simulink model "tricanter_top"  (R2025b)
settings: Solver=FixedStepDiscrete  StartTime=0  StopTime=1500  FixedStep=Ts  RelTol=1e-3
values from neighbouring files (symbols this model uses):
  m0 = 0.0 0.0 0.0 0.0 0.0 0.0 0.0 0.0 0.0 0.0 0.0 0.0 0.0 0.0 0.0 0.0 0.0 0.0 0.0 0.0 0.0 0.0 0.0 0.0 0.0    [tricanter_data.sldd]
  phi0 = 0.0 0.0 0.0 0.0 0.0 0.0 0.0 0.0 0.0 0.0 0.0 0.0 0.0 0.0 0.0 0.0 0.0 0.0 0.0 0.0 0.0 0.0 0.0 0.0 0.0 0.0 0.0 0.0 0.0 0.0 0.0 0.0 0.0 0.0 0.0 0.0 0.0 0.0 0.0 0.0 0.0 0.0 0.0 0.0 0.0 0.0 0.0 0.0 0.0 0.0 0.0 0.0 0.0 0.0 0.0 0.0 0.0 0.0 0.0 0.0 0.0 0.0 0.0 0.0 0.0 0.0 0.0 0.0 0.0 0.0 0.0 0.0 0.0 0.0 0.0 0.0 0.0 0.0 0.0 0.0 0.0 0.0 0.0 0.0 0.0 0.0 0.0 0.0 0.0 0.0 0.0 0.0 0.0 0.0 0.0 0.0 0.0 0.0 0.0 0.0    [tricanter_data.sldd]
  TricInputs0 = 0.03    [tricanter_data.sldd]
  TricParams = 0.04    [tricanter_data.sldd]
  Ts = 1.0    [tricanter_data.sldd]
undefined symbols (not defined in the file or in its folder): DiscIntNeverNeededParam
settings Model: DataDictionary=tricanter_data.sldd  Creator=User  LastModifiedBy=User

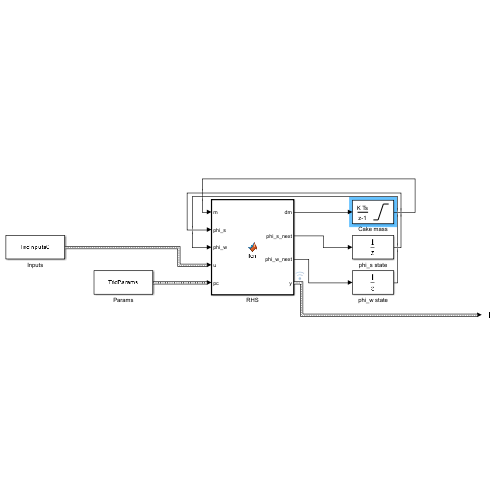
[thumbnail: Simulink's stored preview of the top-level diagram]
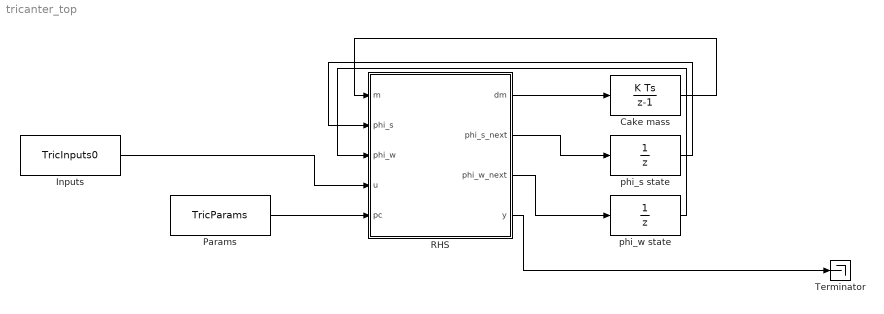
== system tricanter_top ==
  Cake mass : DiscreteIntegrator  InitialCondition=m0  SampleTime=Ts  LimitOutput=on  LowerSaturationLimit=0  ICPrevOutput=DiscIntNeverNeededParam  ICPrevScaledInput=DiscIntNeverNeededParam
  Inputs : Constant  Value=TricInputs0  VectorParams1D=off  OutDataTypeStr=Bus: BusTricInputs
  Params : Constant  Value=TricParams  VectorParams1D=off  OutDataTypeStr=Bus: BusTricParams
  RHS : MATLAB Function  TreatAsAtomicUnit=on
  Terminator : Terminator
  phi_s state : UnitDelay  InitialCondition=phi0  SampleTime=Ts  HasFrameUpgradeWarning=on
  phi_w state : UnitDelay  InitialCondition=phi0  SampleTime=Ts  HasFrameUpgradeWarning=on
  wires:
  Inputs/1 -> RHS/4(u)
  Params/1 -> RHS/5(pc)
  RHS/1(dm) -> Cake mass/1
  RHS/2(phi_s_next) -> phi_s state/1
  RHS/3(phi_w_next) -> phi_w state/1
  RHS/4(y) -> Terminator/1
  Cake mass/1 -> RHS/1(m)
  phi_s state/1 -> RHS/2(phi_s)
  phi_w state/1 -> RHS/3(phi_w)

== matlab function tricanter_top/RHS ==
  data: m input double size=[25 1]; phi_s input double size=[25 40]; phi_w input double size=[25 40]; dm output double size=[25 1]; phi_s_next output double size=[25 40]; phi_w_next output double size=[25 40]; u input Bus: BusTricInputs; y output Bus: BusTricOut; pc input Bus: BusTricParams; Ts parameter double size=1
function [dm, phi_s_next, phi_w_next, y] = fcn(m, phi_s, phi_w, u, pc, Ts)
%#codegen
[dm, phi_s_next, phi_w_next, y] = tric_rhs(m, phi_s, phi_w, u, pc, Ts);
